simulink model "Sprawozdanie3czesc1"  (R2017b)
settings: Solver=VariableStepAuto  StartTime=0.0  StopTime=10.0  RelTol=1e-3
values from neighbouring files (symbols this model uses):
  L = 10    [Sprawozdanie3czesc2.m]
  R = 2    [Sprawozdanie3czesc2.m]
undefined symbols (not defined in the file or in its folder): wl, wr
libraries: simulink x1
settings Model: Creator=marci  LastModifiedBy=marci

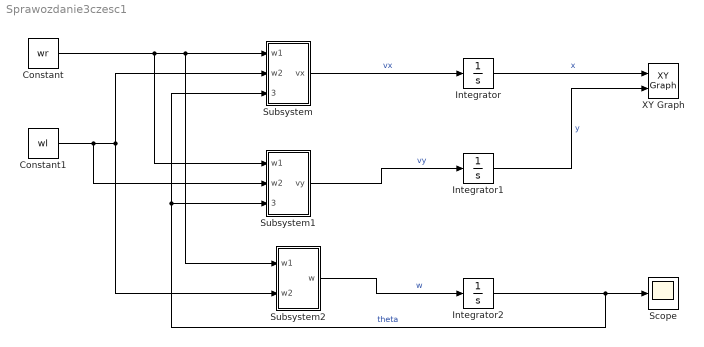
== system Sprawozdanie3czesc1 ==
  Constant : Constant  Value=wr
  Constant1 : Constant  Value=wl
  Integrator : Integrator
  Integrator1 : Integrator
  Integrator2 : Integrator
  Scope : Scope
  Subsystem : Subsystem
  Subsystem1 : Subsystem
  Subsystem2 : Subsystem
  XY Graph : simulink/Sinks/XY Graph  xmin=-1  xmax=1  ymin=-1  ymax=1  st=-1
  wires:
  Constant/1 -> Subsystem1/1(w1), Subsystem/1(w1), Subsystem2/1(w1)
  Constant1/1 -> Subsystem1/2(w2), Subsystem/2(w2), Subsystem2/2(w2)
  Subsystem/1(vx) -> Integrator/1  "vx"
  Integrator/1 -> XY Graph/1  "x"
  Subsystem2/1(w) -> Integrator2/1  "w"
  Integrator2/1 -> Subsystem1/3(theta), Subsystem/3(theta), Scope/1  "theta"
  Subsystem1/1(vy) -> Integrator1/1  "vy"
  Integrator1/1 -> XY Graph/2  "y"

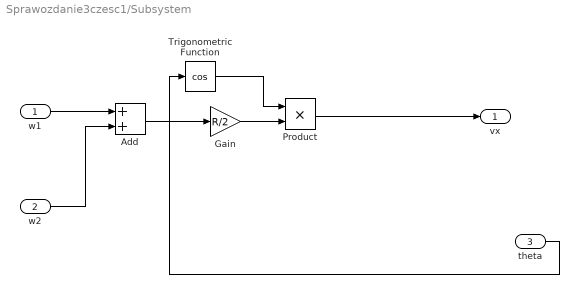
== system Sprawozdanie3czesc1/Subsystem ==
  w1 : Inport
  w2 : Inport  Port=2
  theta : Inport  Port=3
  Add : Sum
  Gain : Gain  Gain=R/2
  Product : Product
  Trigonometric Function : Trigonometry  Operator=cos
  vx : Outport
  wires:
  w1/1 -> Add/1
  Add/1 -> Gain/1
  Product/1 -> vx/1
  theta/1 -> Trigonometric Function/1
  Gain/1 -> Product/2
  w2/1 -> Add/2
  Trigonometric Function/1 -> Product/1

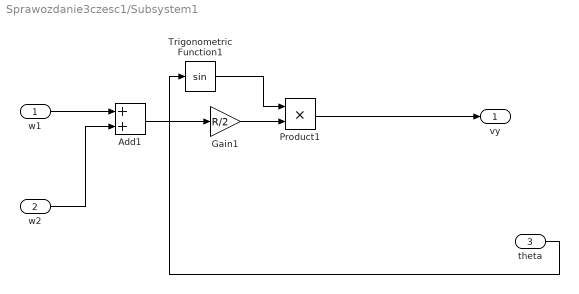
== system Sprawozdanie3czesc1/Subsystem1 ==
  w1 : Inport
  w2 : Inport  Port=2
  theta : Inport  Port=3
  Add1 : Sum
  Gain1 : Gain  Gain=R/2
  Product1 : Product
  Trigonometric Function1 : Trigonometry
  vy : Outport
  wires:
  w1/1 -> Add1/1
  Add1/1 -> Gain1/1
  Product1/1 -> vy/1
  Gain1/1 -> Product1/2
  theta/1 -> Trigonometric Function1/1
  Trigonometric Function1/1 -> Product1/1
  w2/1 -> Add1/2

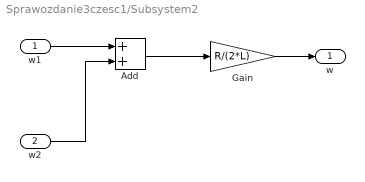
== system Sprawozdanie3czesc1/Subsystem2 ==
  w1 : Inport
  w2 : Inport  Port=2
  Add : Sum
  Gain : Gain  Gain=R/(2*L)
  w : Outport
  wires:
  w1/1 -> Add/1
  Add/1 -> Gain/1
  w2/1 -> Add/2
  Gain/1 -> w/1
